simulink model "23"  (R2021b)
settings: Solver=VariableStepAuto  StartTime=0.0  StopTime=20  RelTol=1e-7
InitFcn:
  | % quadrotor parameters
  | m = 1;
  | C = 1;
  | J_phi = 1;
  | l = 1;
  | J_theta = 1;
  | J_psi = 1;
  | M = blkdiag(1/m,C/J_phi,l/J_theta,l/J_psi);
  | g = 9.81;
  | 
  | % controller parameters
  | kappa = 100;
  | a_1 = 5;
  | a_2 = 10;
  | a_3 = 10;
  | a_4 = 5;
  | a_5 = 1;
  | gamma_1 = 1;
  | gamma_2 = 4;
  | gamma_3 = 6;
  | gamma_4 = 4;
  | L = 5;
  | 
  | ell = 0.9;
settings Model: Creator=olegborisov  LastModifiedBy=antonpyrkin
settings DebuggingCC: UnconnectedInputMsg=none  UnconnectedOutputMsg=none  UnconnectedLineMsg=none
settings ModelReferenceCC: EnableRefExpFcnMdlSchedulingChecks=off
settings RTWCC: DLArmComputeVersion=20.02.1

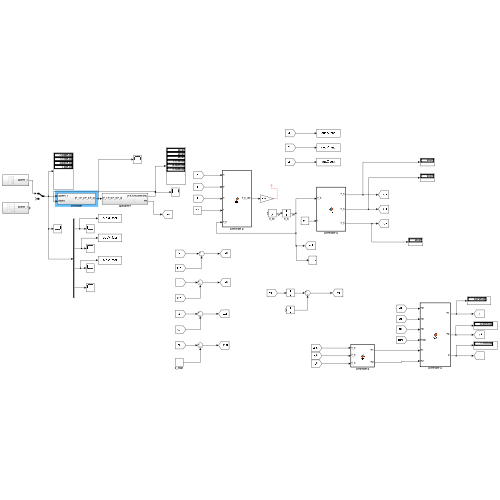
[thumbnail: Simulink's stored preview of the top-level diagram]
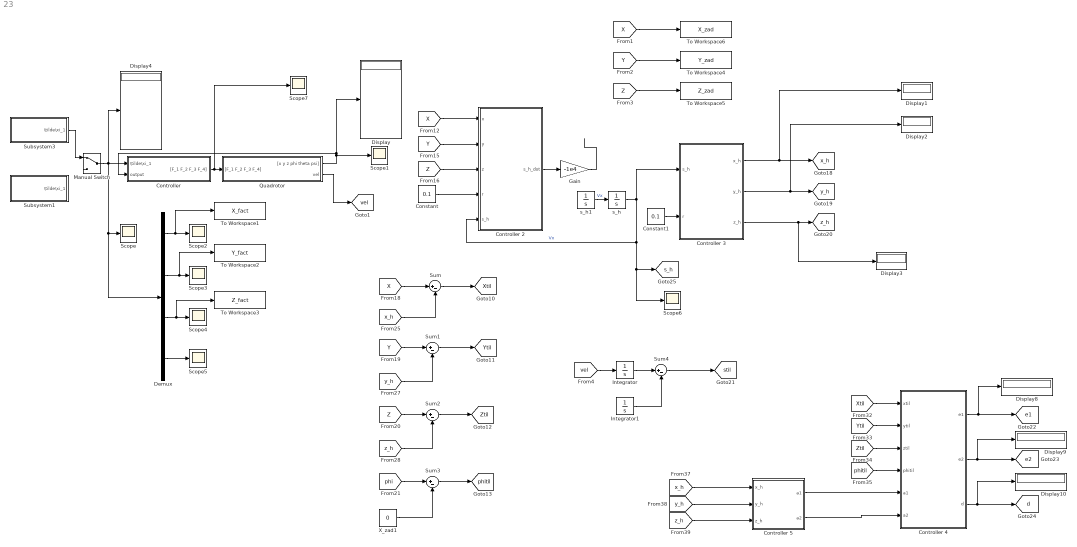
== system 23 ==
  Constant : Constant  Value=0.1
  Constant1 : Constant  Value=0.1
  Controller : Subsystem
  Controller 2 : MATLAB Function  TreatAsAtomicUnit=on
  Controller 3 : MATLAB Function  TreatAsAtomicUnit=on
  Controller 4 : MATLAB Function  TreatAsAtomicUnit=on
  Controller 5 : MATLAB Function  TreatAsAtomicUnit=on
  Demux : Demux
  Display{,1..4,8..10} (8 alike) : Display
  Gain : Gain  Gain=-1e4
  Integrator : Integrator
  Integrator1 : Integrator
  Manual Switch : ManualSwitch
  Quadrotor : Subsystem
  Scope{,1..7} (8 alike) : Scope
  Subsystem1 : Subsystem
  Subsystem3 : Subsystem
  Sum{,1..4} (5 alike) : Sum  Inputs=|+-
  To Workspace1 : ToWorkspace  VariableName=X_fact  SaveFormat=Timeseries  SampleTime=-1
  To Workspace2 : ToWorkspace  VariableName=Y_fact  SaveFormat=Timeseries  SampleTime=-1
  To Workspace3 : ToWorkspace  VariableName=Z_fact  SaveFormat=Timeseries  SampleTime=-1
  To Workspace4 : ToWorkspace  VariableName=Y_zad  SaveFormat=Timeseries  SampleTime=-1
  To Workspace5 : ToWorkspace  VariableName=Z_zad  SaveFormat=Timeseries  SampleTime=-1
  To Workspace6 : ToWorkspace  VariableName=X_zad  SaveFormat=Timeseries  SampleTime=-1
  X_zad1 : Constant  Value=0
  s_h : Integrator  InitialCondition=2/3
  s_h1 : Integrator  InitialCondition=1
  tag scope: Xtil=global, Ytil=global, Ztil=global, d=global, e1=global, e2=global, phitil=global, s_h=global, stil=global, vel=global, x_h=global, y_h=global, z_h=global
  wires:
  Quadrotor/1("[x y z phi theta psi]") -> Display/1, Controller/2(output), Scope1/1
  Manual Switch/1 -> Display4/1, Controller/1(\tilde\xi_1), Demux/1, Scope/1
  Demux/1 -> To Workspace1/1, Scope2/1
  Demux/2 -> To Workspace2/1, Scope3/1
  Demux/4 -> Scope5/1
  Demux/3 -> To Workspace3/1, Scope4/1
  Controller 3/2(y_h) -> Display2/1, [y_h]
  Controller 3/3(z_h) -> Display3/1, [z_h]
  s_h/1 -> Controller 3/1(s_h), Scope6/1, [s_h], Controller 2/5(s_h)  "Vx"
  [Z] -> Controller 2/3(z)
  Constant1/1 -> Controller 3/2(r)
  Gain/1 -> ?
  [Y] -> Controller 2/2(y)
  Constant/1 -> Controller 2/4(r)
  Controller 3/1(x_h) -> Display1/1, [x_h]
  Controller 2/1(s_h_dot) -> Gain/1
  [X] -> Controller 2/1(x)
  [X] -> To Workspace6/1
  [Y] -> To Workspace4/1
  [Z] -> To Workspace5/1
  Controller 4/1(e1) -> [e1], Display8/1
  Controller 5/2(a2) -> Controller 4/6(a2)
  [Xtil] -> Controller 4/1(xtil)
  [z_h] -> Controller 5/3(z_h)
  Controller 5/1(a1) -> Controller 4/5(a1)
  [y_h] -> Controller 5/2(y_h)
  [vel] -> Integrator/1
  [phitil] -> Controller 4/4(phitil)
  Controller 4/2(e2) -> Display9/1, [e2]
  Integrator/1 -> Sum4/1
  [x_h] -> Controller 5/1(x_h)
  Controller 4/3(d) -> Display10/1, [d]
  [Ztil] -> Controller 4/3(ztil)
  [Ytil] -> Controller 4/2(ytil)
  [y_h] -> Sum1/2
  Sum1/1 -> [Ytil]
  Sum3/1 -> [phitil]
  [x_h] -> Sum/2
  X_zad1/1 -> Sum3/2
  [z_h] -> Sum2/2
  [phi] -> Sum3/1
  [Y] -> Sum1/1
  Sum/1 -> [Xtil]
  Sum2/1 -> [Ztil]
  [Z] -> Sum2/1
  [X] -> Sum/1
  Controller/1("[F_1 F_2 F_3 F_4]") -> Scope7/1, Quadrotor/1("[F_1 F_2 F_3 F_4]")
  Quadrotor/2(vel) -> [vel]
  Integrator1/1 -> Sum4/2
  Sum4/1 -> [stil]
  Subsystem3/1(\tilde\xi_1) -> Manual Switch/1
  s_h1/1 -> s_h/1  "Vx"

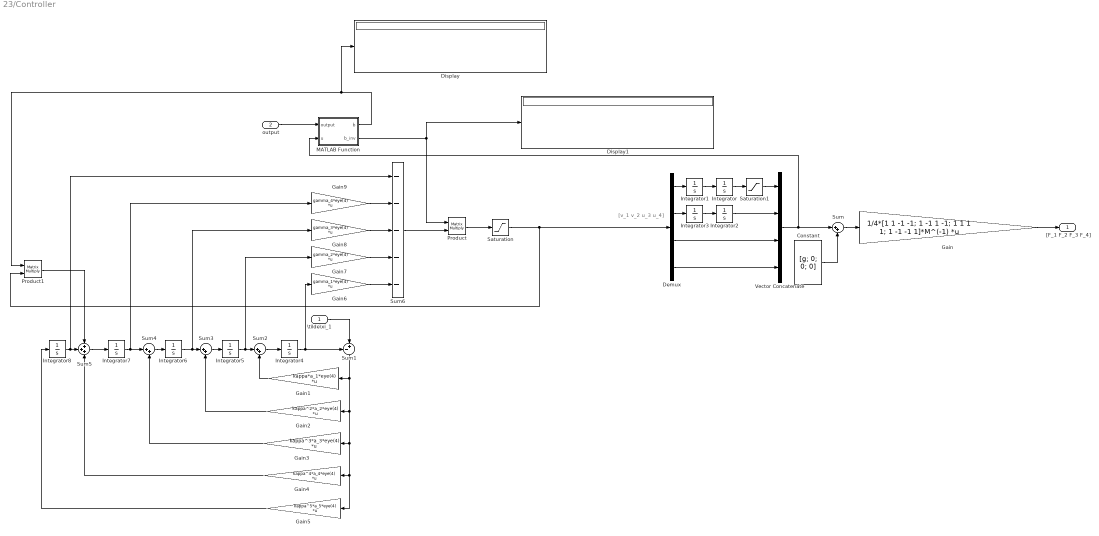
== system 23/Controller ==
  note: [v_1 v_2 u_3 u_4]
  \tilde\xi_1 : Inport
  output : Inport  Port=2
  Constant : Constant  Value=[g; 0; 0; 0]  VectorParams1D=off
  Demux : Demux
  Display : Display
  Display1 : Display
  Gain : Gain  Gain=1/4*[1 1 -1 -1; 1 -1 1 -1; 1 1 1 1; 1 -1 -1 1]*M^(-1)  Multiplication=Matrix(K*u) (u vector)
  Gain1 : Gain  Gain=kappa*a_1*eye(4)  Multiplication=Matrix(K*u) (u vector)
  Gain2 : Gain  Gain=kappa^2*a_2*eye(4)  Multiplication=Matrix(K*u) (u vector)
  Gain3 : Gain  Gain=kappa^3*a_3*eye(4)  Multiplication=Matrix(K*u) (u vector)
  Gain4 : Gain  Gain=kappa^4*a_4*eye(4)  Multiplication=Matrix(K*u) (u vector)
  Gain5 : Gain  Gain=kappa^5*a_5*eye(4)  Multiplication=Matrix(K*u) (u vector)
  Gain6 : Gain  Gain=gamma_1*eye(4)  Multiplication=Matrix(K*u) (u vector)
  Gain7 : Gain  Gain=gamma_2*eye(4)  Multiplication=Matrix(K*u) (u vector)
  Gain8 : Gain  Gain=gamma_3*eye(4)  Multiplication=Matrix(K*u) (u vector)
  Gain9 : Gain  Gain=gamma_4*eye(4)  Multiplication=Matrix(K*u) (u vector)
  Integrator{,1..8} (9 alike) : Integrator
  MATLAB Function : MATLAB Function  TreatAsAtomicUnit=on
  Product : Product  Multiplication=Matrix(*)
  Product1 : Product  Multiplication=Matrix(*)
  Saturation : Saturate  UpperLimit=L  LowerLimit=-L
  Saturation1 : Saturate  UpperLimit=ell*g  LowerLimit=-ell*g
  Sum{,2..4} (4 alike) : Sum  Inputs=|++
  Sum1 : Sum  Inputs=-+|
  Sum5 : Sum  Inputs=+++
  Sum6 : Sum  Inputs=-----
  Vector Concatenate : Concatenate  NumInputs=4
  "[F_1 F_2 F_3 F_4]" : Outport
  wires:
  Gain/1 -> "[F_1 F_2 F_3 F_4]"/1
  Sum/1 -> Gain/1
  Constant/1 -> Sum/2
  Integrator1/1 -> Integrator/1
  Integrator3/1 -> Integrator2/1
  Integrator/1 -> Saturation1/1
  Integrator2/1 -> Vector Concatenate/2
  Demux/1 -> Integrator1/1
  Demux/2 -> Integrator3/1
  Demux/3 -> Vector Concatenate/3
  Demux/4 -> Vector Concatenate/4
  Vector Concatenate/1 -> MATLAB Function/2(u), Sum/1
  Integrator4/1 -> Sum1/1, Gain6/1
  \tilde\xi_1/1 -> Sum1/2
  Sum1/1 -> Gain5/1, Gain4/1, Gain3/1, Gain2/1, Gain1/1
  Gain1/1 -> Sum2/2
  Sum2/1 -> Integrator4/1
  Integrator5/1 -> Gain7/1, Sum2/1
  Sum3/1 -> Integrator5/1
  Gain2/1 -> Sum3/2
  Integrator6/1 -> Gain8/1, Sum3/1
  Sum4/1 -> Integrator6/1
  Gain3/1 -> Sum4/2
  Integrator7/1 -> Gain9/1, Sum4/1
  Sum5/1 -> Integrator7/1
  Gain4/1 -> Sum5/3
  Integrator8/1 -> Sum6/1, Sum5/2
  Gain5/1 -> Integrator8/1
  Gain6/1 -> Sum6/5
  Gain7/1 -> Sum6/4
  Gain8/1 -> Sum6/3
  Gain9/1 -> Sum6/2
  Sum6/1 -> Product/2
  Product/1 -> Saturation/1
  Product1/1 -> Sum5/1
  MATLAB Function/2(b_inv) -> Display1/1, Product/1
  MATLAB Function/1(b) -> Product1/1, Display/1
  output/1 -> MATLAB Function/1(output)
  Saturation/1 -> Product1/2, Demux/1
  Saturation1/1 -> Vector Concatenate/1

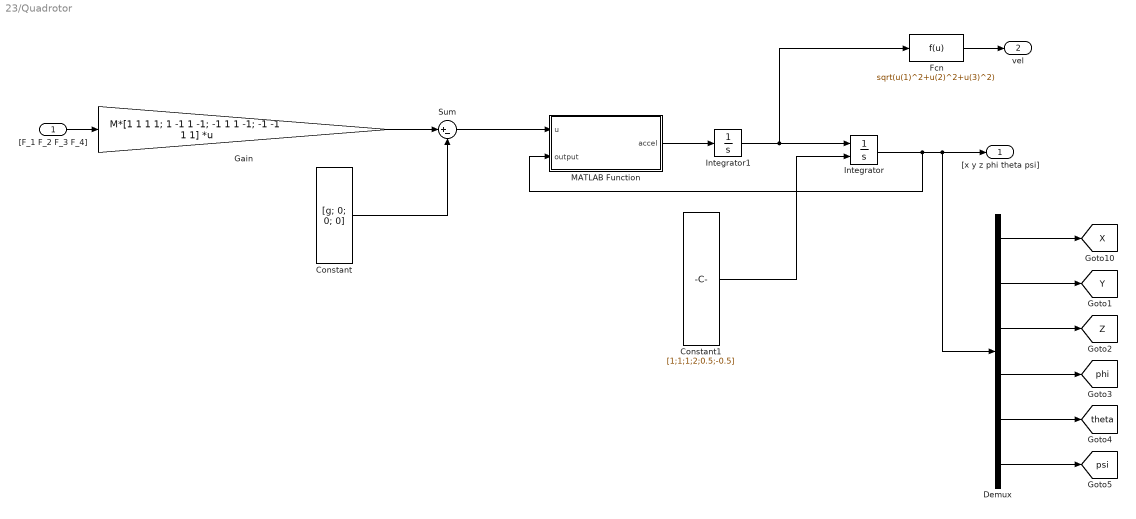
== system 23/Quadrotor ==
  "[F_1 F_2 F_3 F_4]" : Inport
  Constant : Constant  Value=[g; 0; 0; 0]  VectorParams1D=off
  Constant1 : Constant  Value=[1;1;1;2;0.5;-0.5]  VectorParams1D=off
  Demux : Demux  Outputs=6
  Fcn : Fcn  Expr=sqrt(u(1)^2+u(2)^2+u(3)^2)
  Gain : Gain  Gain="M*[1 1 1 1; 1 -1 1 -1; -1 1 1 -1;  -1 -1 1 1]"  Multiplication=Matrix(K*u) (u vector)
  Integrator : Integrator  InitialConditionSource=external  InitialCondition=[0;1;1;1;0;0]
  Integrator1 : Integrator
  MATLAB Function : MATLAB Function  TreatAsAtomicUnit=on
  Sum : Sum  Inputs=|+-
  "[x y z phi theta psi]" : Outport
  vel : Outport  Port=2
  tag scope: X=global, Y=global, Z=global, phi=global, psi=global, theta=global
  wires:
  Integrator1/1 -> Fcn/1, Integrator/1
  Integrator/1 -> Demux/1, "[x y z phi theta psi]"/1, MATLAB Function/2(output)
  MATLAB Function/1(accel) -> Integrator1/1
  "[F_1 F_2 F_3 F_4]"/1 -> Gain/1
  Gain/1 -> Sum/1
  Constant/1 -> Sum/2
  Sum/1 -> MATLAB Function/1(u)
  Constant1/1 -> Integrator/2
  Demux/1 -> [X]
  Demux/2 -> [Y]
  Demux/3 -> [Z]
  Demux/4 -> [phi]
  Demux/5 -> [theta]
  Demux/6 -> [psi]
  Fcn/1 -> vel/1

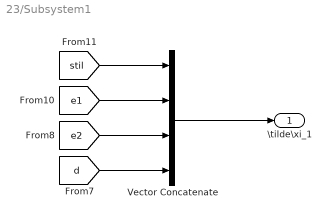
== system 23/Subsystem1 ==
  Vector Concatenate : Concatenate  NumInputs=4
  \tilde\xi_1 : Outport
  wires:
  [e1] -> Vector Concatenate/2
  [stil] -> Vector Concatenate/1
  [e2] -> Vector Concatenate/3
  Vector Concatenate/1 -> \tilde\xi_1/1
  [d] -> Vector Concatenate/4

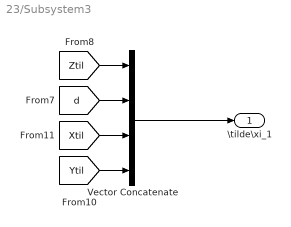
== system 23/Subsystem3 ==
  Vector Concatenate : Concatenate  NumInputs=4
  \tilde\xi_1 : Outport
  wires:
  Vector Concatenate/1 -> \tilde\xi_1/1
  [Ztil] -> Vector Concatenate/1
  [d] -> Vector Concatenate/2
  [Xtil] -> Vector Concatenate/3
  [Ytil] -> Vector Concatenate/4

== matlab function 23/Controller/MATLAB Function ==
  data: output input; u input; b output; b_inv output
function [b,b_inv] = fcn(output,u)

no = 0;
simple = 1;
full = 2;

flag = full;

phi = output(4);

theta = output(5);

psi = output(6);

ct = cos(theta);
st = sin(theta);

cp = cos(psi);
sp = sin(psi);

g = 9.81;
d = u(1)+g;

if flag == simple
b = [1 0 0 0; 
     0 1 0 0; 
     0 0 cos(phi)*d sin(phi)*d; 
     0 0 sin(phi)*d -cos(phi)*d];
elseif flag == full
b = [1 0 0 0; 
     0 1 0 0; 
     0 0 cos(phi) -sin(phi); 
     0 0 sin(phi) cos(phi)]*...
    [ct*cp 0 -st*cp*d -ct*sp*d ; 
     0 1 0 0;
     st*cp 0 ct*cp*d -st*sp*d;
     -sp 0 0 -cp*d];
else 
    b =eye(4);
end

b_inv  = inv(b);

== matlab function 23/Quadrotor/MATLAB Function ==
  data: u input; accel output; output input
function accel = fcn(u, output)

g = 9.81;
phi = output(4);
theta = output(5);
psi = output(6);

accel_lin = [cos(phi)*sin(theta)*cos(psi)+sin(phi)*sin(psi);...
    sin(phi)*sin(theta)*cos(psi)-cos(phi)*sin(psi);...
    cos(theta)*cos(psi)]*(u(1)+g)-[0; 0; g];

accel_ang = [u(2); u(3); u(4)];

accel = [accel_lin; accel_ang];

== matlab function 23/Controller 2 ==
  data: x input; y input; z input; r input; s_h_dot output; s_h input
function s_h_dot   = fcn(x,y,z,r,s_h)


rho = 1;
H = 3*s_h - x - y - z;

%rho = 1 + r*cos(s_h)*x + r*sin(s_h)*y;

%H = r*sin(s_h)*x - r*cos(s_h)*y - z + s_h;

s_h_dot = rho*H;

== matlab function 23/Controller 3 ==
  data: s_h input; r input; x_h output; y_h output; z_h output
function [x_h,y_h,z_h]   = fcn(s_h, r)


x_h = s_h;

y_h = s_h;

z_h = s_h;

%x_h = r * cos(s_h);

%y_h = r* sin(s_h);

%z_h = s_h;

== matlab function 23/Controller 4 ==
  data: xtil input; ytil input; ztil input; phitil input; a1 input; a2 input; e1 output; e2 output; d output
function [e1,e2,d]   = fcn(xtil,ytil,ztil,phitil,a1,a2)

xyztil = [xtil;ytil;ztil];

e1 = [-sin(a1); cos(a1); 0]'*xyztil;

e2 = [cos(a1)*sin(a2); sin(a1)*sin(a2); cos(a2)]'*xyztil;

d = phitil;

== matlab function 23/Controller 5 ==
  data: x_h input; y_h input; a1 output; a2 output; z_h input
function [a1,a2]   = fcn(x_h,y_h,z_h)


a1 = atan2(y_h, - x_h);

a2 = -pi/4;
